simulink model "PTC"  (R2016a)
settings: Solver=VariableStepAuto  StartTime=0.0  StopTime=10  RelTol=1e-3
libraries: fl_lib x11, nesl_utility x11, elec_lib x3
settings Model: Creator=enes_  LastModifiedBy=enes_

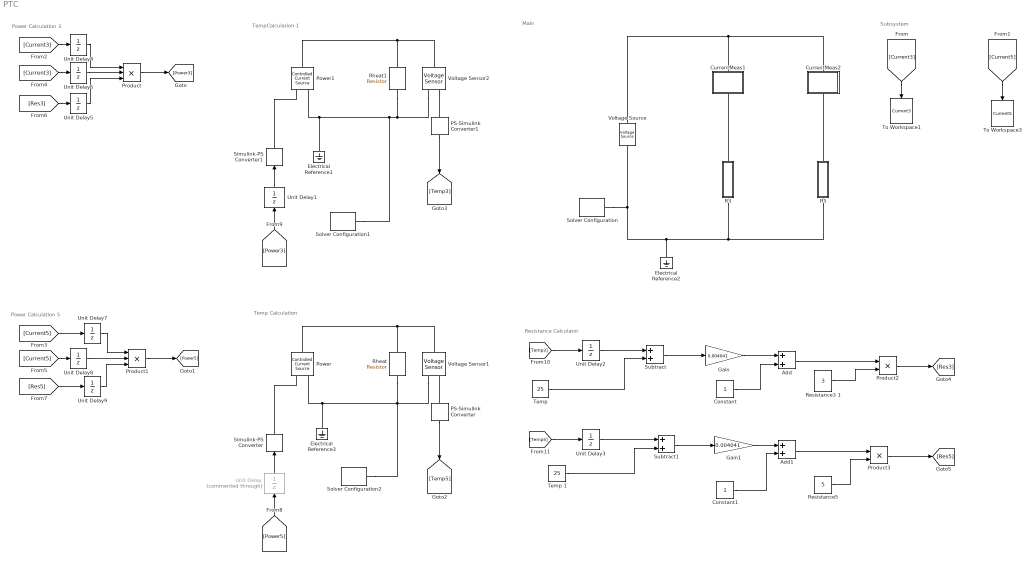
== system PTC ==
  note: TempCalcularion
      | 1
  note: Temp Calculation
  note: Subsystem
  note: Main
  note: Resistance Calculator
  note: Power Calculation 5
  note: Power Calculation 3
  Add : Sum
  Add1 : Sum
  Constant : Constant
  Constant1 : Constant
  CurrentMeas1 : Subsystem
  CurrentMeas2 : Subsystem
  Electrical Reference1 : fl_lib/Electrical/Electrical Elements/Electrical Reference
  Electrical Reference2 : fl_lib/Electrical/Electrical Elements/Electrical Reference
  Electrical Reference3 : fl_lib/Electrical/Electrical Elements/Electrical Reference
  Gain : Gain  Gain=0.004041
  Gain1 : Gain  Gain=0.004041
  PS-Simulink Converter : nesl_utility/PS-Simulink Converter  PhysicalDomain=network_engine_domain  SubClassName=ps_output  LeftPortType=input  RightPortType=output  PseudoPeriodic=off  Frequencies=[]  Unit=1  AffineConversion=off
  PS-Simulink Converter1 : nesl_utility/PS-Simulink Converter  PhysicalDomain=network_engine_domain  SubClassName=ps_output  LeftPortType=input  RightPortType=output  PseudoPeriodic=off  Frequencies=[]  Unit=1  AffineConversion=off
  Power : fl_lib/Electrical/Electrical Sources/Controlled Current Source
  Power1 : fl_lib/Electrical/Electrical Sources/Controlled Current Source
  Product : Product  Inputs=3
  Product1 : Product  Inputs=3
  Product2 : Product
  Product3 : Product
  R3 : Subsystem
  R5 : Subsystem
  Resistance3 1 : Constant  Value=3
  Resistance5 : Constant  Value=5
  Rheat : elec_lib/Passive Devices/Resistor  R=0.5 Ohm  R_tol=5  enable_R_tol=0  tol_distribution=1  nSigma=4  enable_operating_limits=0  operating_limit_action=2  max_working_voltage=100 V  power_rating=1 W  enable_faults=0  fault_action=1  R_faulted=Inf Ohm  enable_temporal_fault=0  t_fault=1 s  enable_behavioral_fault=0  max_permissible_current=1 A  t_fail_on_current=1 s  noise_mode=0  sample_time=0.001 s  repeatability=1  auto_seed=4177890155  user_seed=0  Tdevice=25 degC  alpha=0.00393 1/K  Tmeas=25 degC  thermal_mass=100 J/K  initial_temperature=25 degC  power_derating_T1=70 degC  power_derating_T2=155 degC  operating_temperature_range_vec=[ -50 150 ] degC
  Rheat1 : elec_lib/Passive Devices/Resistor  R=0.5 Ohm  R_tol=5  enable_R_tol=0  tol_distribution=1  nSigma=4  enable_operating_limits=0  operating_limit_action=2  max_working_voltage=100 V  power_rating=1 W  enable_faults=0  fault_action=1  R_faulted=Inf Ohm  enable_temporal_fault=0  t_fault=1 s  enable_behavioral_fault=0  max_permissible_current=1 A  t_fail_on_current=1 s  noise_mode=0  sample_time=0.001 s  repeatability=1  auto_seed=549817661  user_seed=0  Tdevice=25 degC  alpha=0.00393 1/K  Tmeas=25 degC  thermal_mass=100 J/K  initial_temperature=25 degC  power_derating_T1=70 degC  power_derating_T2=155 degC  operating_temperature_range_vec=[ -50 150 ] degC
  Simulink-PS Converter : nesl_utility/Simulink-PS Converter  PhysicalDomain=network_engine_domain  SubClassName=ps_input  LeftPortType=input  RightPortType=output  PseudoPeriodic=off  Frequencies=[]  NoiseDistribution=none  NoiseParameters=[]  Unit=1  AffineConversion=off  InputFiltering=off  SimscapeFilterOrder=1  InputFilterTimeConstant=0.001  UdotUserProvided=1
  Simulink-PS Converter1 : nesl_utility/Simulink-PS Converter  PhysicalDomain=network_engine_domain  SubClassName=ps_input  LeftPortType=input  RightPortType=output  PseudoPeriodic=off  Frequencies=[]  NoiseDistribution=none  NoiseParameters=[]  Unit=1  AffineConversion=off  InputFiltering=off  SimscapeFilterOrder=1  InputFilterTimeConstant=0.001  UdotUserProvided=1
  Solver Configuration : nesl_utility/Solver Configuration  PhysicalDomain=network_engine_domain  SubClassName=solver  LeftPortType=input  RightPortType=generic  Accelerate=off  Tones=[]  Harmonics=[]  SimulateNoise=off  Profile=off  UseLocalSampling=off  EnableSwitchedLinearOptims=on  FrequencyDomain=off  UseCCode=off  RelTol=0.001  AbsTol=1e-06  MinStep=1e-09  ToWorkspace=off  RevertToSquareIcSolve=off  NumHomotopyIterations=100  PhasorMode=off  PhasorModeNumHarmonics=1  OverrideAbsTol=off  DoDC=off  ResidualTolerance=1e-09  UseLocalSolver=off  LocalSolverChoice=NE_BACKWARD_EULER_ADVANCER  LocalSolverSampleTime=0.001  DoFixedCost=off  MaxNonlinIter=3  MaxModeIter=2  LinearAlgebra=Sparse  DelaysMemoryBudget=1024  AutomaticFiltering=on  FilteringTimeConstant=0.001
  Solver Configuration1 : nesl_utility/Solver Configuration  PhysicalDomain=network_engine_domain  SubClassName=solver  LeftPortType=input  RightPortType=generic  Accelerate=off  Tones=[]  Harmonics=[]  SimulateNoise=off  Profile=off  UseLocalSampling=off  EnableSwitchedLinearOptims=on  FrequencyDomain=off  UseCCode=off  RelTol=0.001  AbsTol=1e-06  MinStep=1e-09  ToWorkspace=off  RevertToSquareIcSolve=off  NumHomotopyIterations=100  PhasorMode=off  PhasorModeNumHarmonics=1  OverrideAbsTol=off  DoDC=off  ResidualTolerance=1e-09  UseLocalSolver=off  LocalSolverChoice=NE_BACKWARD_EULER_ADVANCER  LocalSolverSampleTime=0.001  DoFixedCost=off  MaxNonlinIter=3  MaxModeIter=2  LinearAlgebra=Sparse  DelaysMemoryBudget=1024  AutomaticFiltering=on  FilteringTimeConstant=0.001
  Solver Configuration2 : nesl_utility/Solver Configuration  PhysicalDomain=network_engine_domain  SubClassName=solver  LeftPortType=input  RightPortType=generic  Accelerate=off  Tones=[]  Harmonics=[]  SimulateNoise=off  Profile=off  UseLocalSampling=off  EnableSwitchedLinearOptims=on  FrequencyDomain=off  UseCCode=off  RelTol=0.001  AbsTol=1e-06  MinStep=1e-09  ToWorkspace=off  RevertToSquareIcSolve=off  NumHomotopyIterations=100  PhasorMode=off  PhasorModeNumHarmonics=1  OverrideAbsTol=off  DoDC=off  ResidualTolerance=1e-09  UseLocalSolver=off  LocalSolverChoice=NE_BACKWARD_EULER_ADVANCER  LocalSolverSampleTime=0.001  DoFixedCost=off  MaxNonlinIter=3  MaxModeIter=2  LinearAlgebra=Sparse  DelaysMemoryBudget=1024  AutomaticFiltering=on  FilteringTimeConstant=0.001
  Subtract : Sum
  Subtract1 : Sum
  "Temp " : Constant  Value=25
  Temp 1 : Constant  Value=25
  To Workspace1 : ToWorkspace  VariableName=Current3  SaveFormat=Timeseries  SampleTime=-1
  To Workspace3 : ToWorkspace  VariableName=Current5  SaveFormat=Timeseries  SampleTime=-1
  Unit Delay : UnitDelay  Commented=through  SampleTime=-1
  Unit Delay{1..9} (9 alike) : UnitDelay  SampleTime=-1
  Voltage Sensor1 : fl_lib/Electrical/Electrical Sensors/Voltage Sensor
  Voltage Sensor2 : fl_lib/Electrical/Electrical Sensors/Voltage Sensor
  Voltage Source : elec_lib/Sources/Voltage Source  dc_voltage=200 V  ac_voltage=0 V  ac_shift=0 deg  ac_frequency=60 Hz  noise_mode=0  PSD=0 V^2/Hz  sample_time=0.001 s  repeatability=1  auto_seed=3054648517  user_seed=0
  wires:
  [Current3] -> Unit Delay6/1
  [Current3] -> Unit Delay4/1
  Product/1 -> [Power3]
  [Res3] -> Unit Delay5/1
  [Current5] -> Unit Delay8/1
  [Current5] -> Unit Delay7/1
  [Res5] -> Unit Delay9/1
  Product1/1 -> [Power5]
  [Temp5] -> Unit Delay3/1
  "Temp "/1 -> Subtract/2
  Add1/1 -> Product3/1
  Constant/1 -> Add/2
  Constant1/1 -> Add1/2
  Temp 1/1 -> Subtract1/2
  Resistance3 1/1 -> Product2/2
  Gain1/1 -> Add1/1
  Add/1 -> Product2/1
  Product2/1 -> [Res3]
  Gain/1 -> Add/1
  Subtract1/1 -> Gain1/1
  Subtract/1 -> Gain/1
  Product3/1 -> [Res5]
  Resistance5/1 -> Product3/2
  Unit Delay2/1 -> Subtract/1
  [Temp3] -> Unit Delay2/1
  Unit Delay3/1 -> Subtract1/1
  Unit Delay4/1 -> Product/1
  Unit Delay5/1 -> Product/3
  Unit Delay6/1 -> Product/2
  Unit Delay7/1 -> Product1/1
  Unit Delay8/1 -> Product1/2
  Unit Delay9/1 -> Product1/3
  [Current5] -> To Workspace3/1
  [Current3] -> To Workspace1/1
  Unit Delay/1 -> Simulink-PS Converter/1
  PS-Simulink Converter/1 -> [Temp5]
  [Power5] -> Unit Delay/1
  Unit Delay1/1 -> Simulink-PS Converter1/1
  PS-Simulink Converter1/1 -> [Temp3]
  [Power3] -> Unit Delay1/1
  connections:
  R3/RConn1 -- CurrentMeas1/RConn1
  CurrentMeas1/LConn1 -- CurrentMeas2/LConn1 -- Voltage Source/LConn1
  R5/RConn1 -- CurrentMeas2/RConn1
  R5/LConn1 -- R3/LConn1 -- Electrical Reference2/LConn1 -- Solver Configuration/RConn1 -- Voltage Source/RConn1
  Power/LConn1 -- Rheat/LConn1 -- Voltage Sensor1/LConn1
  Simulink-PS Converter/RConn1 -- Power/RConn1
  PS-Simulink Converter/LConn1 -- Voltage Sensor1/RConn1
  Power1/LConn1 -- Voltage Sensor2/LConn1 -- Rheat1/LConn1
  Simulink-PS Converter1/RConn1 -- Power1/RConn1
  PS-Simulink Converter1/LConn1 -- Voltage Sensor2/RConn1
  Voltage Sensor2/RConn2 -- Rheat1/RConn1 -- Solver Configuration1/RConn1 -- Electrical Reference1/LConn1 -- Power1/RConn2
  Solver Configuration2/RConn1 -- Electrical Reference3/LConn1 -- Power/RConn2 -- Voltage Sensor1/RConn2 -- Rheat/RConn1

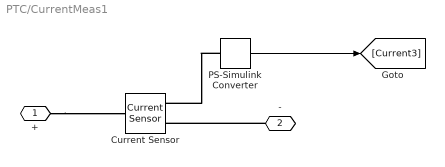
== system PTC/CurrentMeas1 ==
  Current Sensor : fl_lib/Electrical/Electrical Sensors/Current Sensor
  PS-Simulink Converter : nesl_utility/PS-Simulink Converter  PhysicalDomain=network_engine_domain  SubClassName=ps_output  LeftPortType=input  RightPortType=output  PseudoPeriodic=off  Frequencies=[]  Unit=1  AffineConversion=off
  + : PMIOPort  Port=1  Side=Left
  - : PMIOPort  Port=2  Side=Right
  wires:
  PS-Simulink Converter/1 -> [Current3]
  connections:
  +/RConn1 -- Current Sensor/LConn1
  PS-Simulink Converter/LConn1 -- Current Sensor/RConn1
  -/RConn1 -- Current Sensor/RConn2

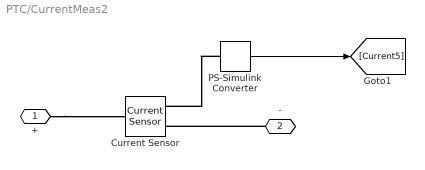
== system PTC/CurrentMeas2 ==
  Current Sensor : fl_lib/Electrical/Electrical Sensors/Current Sensor
  PS-Simulink Converter : nesl_utility/PS-Simulink Converter  PhysicalDomain=network_engine_domain  SubClassName=ps_output  LeftPortType=input  RightPortType=output  PseudoPeriodic=off  Frequencies=[]  Unit=1  AffineConversion=off
  + : PMIOPort  Port=1  Side=Left
  - : PMIOPort  Port=2  Side=Right
  wires:
  PS-Simulink Converter/1 -> [Current5]
  connections:
  +/RConn1 -- Current Sensor/LConn1
  PS-Simulink Converter/LConn1 -- Current Sensor/RConn1
  -/RConn1 -- Current Sensor/RConn2

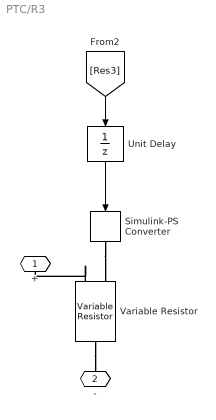
== system PTC/R3 ==
  Simulink-PS Converter : nesl_utility/Simulink-PS Converter  PhysicalDomain=network_engine_domain  SubClassName=ps_input  LeftPortType=input  RightPortType=output  PseudoPeriodic=off  Frequencies=[]  NoiseDistribution=none  NoiseParameters=[]  Unit=1  AffineConversion=off  InputFiltering=off  SimscapeFilterOrder=1  InputFilterTimeConstant=0.001  UdotUserProvided=1
  Unit Delay : UnitDelay  SampleTime=-1
  Variable Resistor : fl_lib/Electrical/Electrical Elements/Variable Resistor  Rmin=0 Ohm  i_specify=off  i_priority=None  i=0 A  v_specify=off  v_priority=None  v=0 V
  + : PMIOPort  Port=1  Side=Right
  - : PMIOPort  Port=2  Side=Left
  wires:
  [Res3] -> Unit Delay/1
  Unit Delay/1 -> Simulink-PS Converter/1
  connections:
  Variable Resistor/LConn2 -- +/RConn1
  Simulink-PS Converter/RConn1 -- Variable Resistor/LConn1
  Variable Resistor/RConn1 -- -/RConn1

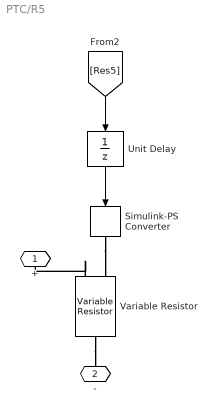
== system PTC/R5 ==
  Simulink-PS Converter : nesl_utility/Simulink-PS Converter  PhysicalDomain=network_engine_domain  SubClassName=ps_input  LeftPortType=input  RightPortType=output  PseudoPeriodic=off  Frequencies=[]  NoiseDistribution=none  NoiseParameters=[]  Unit=1  AffineConversion=off  InputFiltering=off  SimscapeFilterOrder=1  InputFilterTimeConstant=0.001  UdotUserProvided=1
  Unit Delay : UnitDelay  SampleTime=-1
  Variable Resistor : fl_lib/Electrical/Electrical Elements/Variable Resistor  Rmin=0 Ohm  i_specify=off  i_priority=None  i=0 A  v_specify=off  v_priority=None  v=0 V
  + : PMIOPort  Port=1  Side=Right
  - : PMIOPort  Port=2  Side=Left
  wires:
  [Res5] -> Unit Delay/1
  Unit Delay/1 -> Simulink-PS Converter/1
  connections:
  Variable Resistor/LConn2 -- +/RConn1
  Simulink-PS Converter/RConn1 -- Variable Resistor/LConn1
  Variable Resistor/RConn1 -- -/RConn1
